simulink subsystem "MagDipole"  (R2021a)
settings: Solver=VariableStepAuto  StartTime=0.0  StopTime=10.0  RelTol=1e-3
undefined symbols (not defined in the file): B0, RE
settings Model: Creator=Laura  LastModifiedBy=Laura

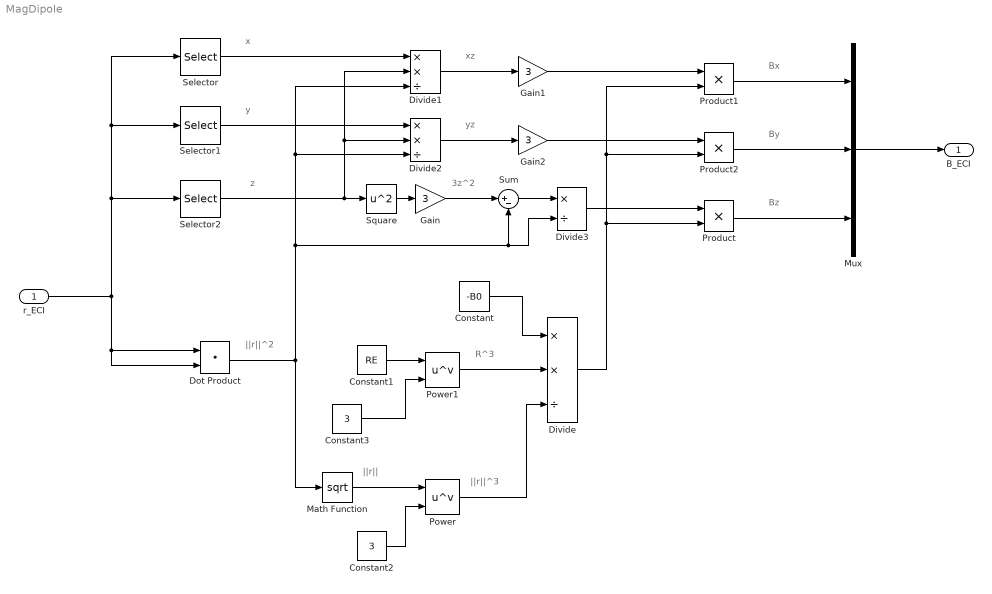
== system MagDipole ==
  note: z
  note: x
  note: y
  note: R^3
  note: ||r||^2
  note: xz
  note: By
  note: ||r||
  note: yz
  note: 3z^2
  note: ||r||^3
  note: Bz
  note: Bx
  r_ECI : Inport
  Constant : Constant  Value=-B0
  Constant1 : Constant  Value=RE
  Constant2 : Constant  Value=3
  Constant3 : Constant  Value=3
  Divide : Product  Inputs=**/
  Divide1 : Product  Inputs=**/
  Divide2 : Product  Inputs=**/
  Divide3 : Product  Inputs=*/
  Dot Product : DotProduct  InputSameDT=on  OutDataTypeStr=Inherit: Inherit via internal rule
  Gain : Gain  Gain=3
  Gain1 : Gain  Gain=3
  Gain2 : Gain  Gain=3
  Math Function : Math  Operator=sqrt  SignedPower=on  SaturateOnIntegerOverflow=on
  Mux : Mux  Inputs=3
  Power : Math  Operator=pow  SaturateOnIntegerOverflow=on
  Power1 : Math  Operator=pow  SaturateOnIntegerOverflow=on
  Product : Product
  Product1 : Product
  Product2 : Product
  Selector : Selector  InputPortWidth=3  IndexOptions=Index vector (dialog)  Indices=[1]  OutputSizes=1
  Selector1 : Selector  InputPortWidth=3  IndexOptions=Index vector (dialog)  Indices=[2]  OutputSizes=1
  Selector2 : Selector  InputPortWidth=3  IndexOptions=Index vector (dialog)  Indices=[3]  OutputSizes=1
  Square : Math  Operator=square  SaturateOnIntegerOverflow=on
  Sum : Sum  Inputs=|+-
  B_ECI : Outport
  wires:
  Constant1/1 -> Power1/1
  Product1/1 -> Mux/1
  Power1/1 -> Divide/2
  Dot Product/1 -> Divide3/2, Sum/2, Divide1/3, Divide2/3, Math Function/1
  Power/1 -> Divide/3
  Divide/1 -> Product/2, Product1/2, Product2/2
  Square/1 -> Gain/1
  Constant3/1 -> Power1/2
  Constant/1 -> Divide/1
  Product2/1 -> Mux/2
  Product/1 -> Mux/3
  Mux/1 -> B_ECI/1
  Divide2/1 -> Gain2/1
  Divide1/1 -> Gain1/1
  Math Function/1 -> Power/1
  Divide3/1 -> Product/1
  Selector1/1 -> Divide2/1
  r_ECI/1 -> Dot Product/2, Dot Product/1, Selector/1, Selector1/1, Selector2/1
  Gain2/1 -> Product2/1
  Constant2/1 -> Power/2
  Selector2/1 -> Divide1/2, Divide2/2, Square/1
  Selector/1 -> Divide1/1
  Gain1/1 -> Product1/1
  Gain/1 -> Sum/1
  Sum/1 -> Divide3/1
